simulink model "MPC View 3D"  (R2025b)
settings: Solver=VariableStepAuto  StartTime=0.0  StopTime=15  RelTol=1e-3
values from neighbouring files (symbols this model uses):
  sys_c = ss(A, B, C, D,      'StateName',  {'Angulo (rad)', 'Velocidad (rad/s)'},      'InputName',  {'Torque (Nm)'},      'OutputName', {'Angulo (rad)'})    [Modelo.m]
libraries: simulink x2, autolibshared x1, mpclib x1, sim3dlib x1, sim3dautolib x1
settings Model: Creator=Camilo  LastModifiedBy=Camilo

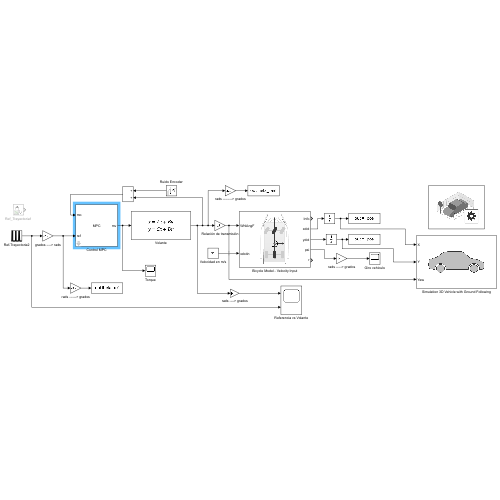
[thumbnail: Simulink's stored preview of the top-level diagram]
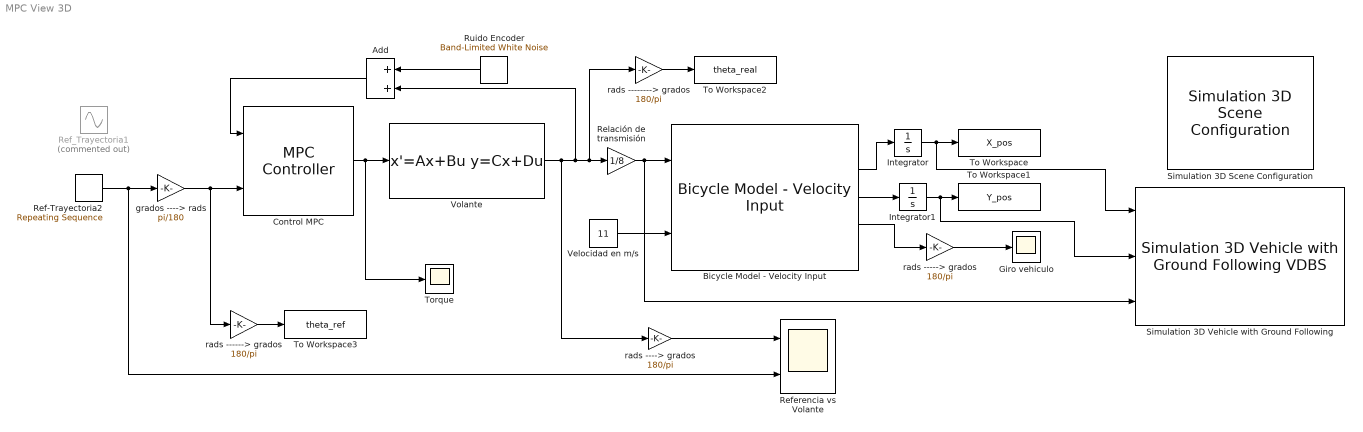
== system MPC View 3D ==
  Add : Sum
  Bicycle Model - Velocity Input : autolibshared/Bicycle Model - Velocity Input  trackMode=Single (bicycle)  inputMode=External longitudinal velocity  frontSteerMode=on  rearSteerMode=off  windMode=off  muMode=off  extFMode=off  extMMode=off  aMode=3  NF=2  NR=2  m=2000  a=1.4  b=1.6  h=0.35  X_o=0  xdot_o=0  CalphaMode=off  sigmaMode=on  w=[1.4,1.4]  Cy_f=12e3  Cy_r=11e3  sigma_f=.1  sigma_r=.1  alpha_f_brk=[-.1 .1]  Cy_f_data=[-9e3 9e3]  alpha_r_brk=[-.1 .1]  Cy_r_data=[-9e3 9e3]  Y_o=0  ydot_o=0  Izz=4000  psi_o=0  r_o=0  Af=2  Cd=.3  Cl=.1  Cpm=.1  beta_w=[0 0.01:0.01:0.3]  Cs=[0 0.01:0.01:0.3]  Cym=[0 1e-6:0.01:0.3]  Pabs=101325  Tair=273  g=9.81  mu=1  xdot_tol=.01  Fznom=5000  Fxtire_sat=1e6  Fytire_sat=1e6  longOff=0  latOff=0  vertOff=0
      settings: LibrarySourceBlock=drivingscenarioandsensors/Bicycle Model - Velocity Input
  Control MPC : mpclib/MPC Controller  SCDEnableBlockLinearizationSpecification=on  mpcobj=mpc1  is_multiple=0  enable_value=0  return_u0=off  updateMPCinCallerWorkspace=on  md_inport=off  mv_inport=off  uref_inport=off  return_cost=off  return_mvseq=off  return_qpstatus=off  return_xseq=off  return_state=off  return_ovseq=off  state_inport=off  umin_inport=off  umax_inport=off  ymin_inport=off  ymax_inport=off  cc_inport=off  ywt_inport=off  uwt_inport=off  duwt_inport=off  rhoeps_inport=off  pm_inport=off  MaximumP=10  HorizonChoice=FixedHorizon  n_ts=0.01  n_p=150  n_mv=1  n_md=0  n_ud=0  n_mo=1  n_uo=0  BlockDataType=double  SampleTimeInherited=off  switch_inport=off
  Giro vehiculo : Scope
      settings: ActiveDisplayYMinimum=-8.075462786158182  ActiveDisplayYMaximum=72.438098994983108
  Integrator : Integrator
  Integrator1 : Integrator
  Ref-Trayectoria2 : simulink/Sources/Repeating Sequence  rep_seq_t=[0, 3, 5, 7, 9, 25]  rep_seq_y=[0, 0, 30, 30, 0, 0]
  Ref_Trayectoria1 : Sin  Commented=on  Amplitude=20  Frequency=0.3  SampleTime=0.01
  Referencia vs Volante : Scope  NumInputPorts=2
      settings: ActiveDisplayYMinimum=-4.394916415083765  ActiveDisplayYMaximum=33.821657379453754  DataLoggingVariableName=ScopeData2
  Relación de transmisión : Gain  Gain=1/8
  Ruido Encoder : simulink/Sources/Band-Limited White Noise  Cov=0.000001  Ts=0.01  seed=[23341]
  Simulation 3D Scene Configuration : sim3dlib/Simulation 3D Scene Configuration  Priority=0  ProjectFormat=Default Scenes  SceneDesc=Double lane change  ProjectName=C:\Program Files\MATLAB\R2025b\toolbox\shared\sim3d_projects\automotive_project_windows\UE\WindowsNoEditor\VehicleSimulation.exe  ScenePath=/Game/Maps/HwStrght  EnableOpenDRIVE=off  vehTagList={'Custom';'Scene Origin';'SimulinkVehicle1'}  vehTag=SimulinkVehicle1  AttachedCameraRelativeTranslation=[0 0 0]  FreeCameraDefaultInitialTranslation=[-6, 0, 2]  AttachedCameraRelativeRotation=[0 0 0]  FreeCameraDefaultInitialRotation=[0, -15, 0]  ViewpointName=Custom  FreeCameraInitialTranslation=[0 0 0]  ViewpointTranslation=[0 0 0]  FreeCameraInitialRotation=[0 0 0]  ViewpointRotation=[0 0 0]  OpVisEn=off  Ts=.01  EnableWindow=on  EnableRemoteAccess=off  EnableWeather=off  SunAzimuth=90  SunAltitude=40.0  EnableGeospatialSun=off  Latitude=0  Longitude=0  Date=2023-01-01  Time=10:30:00  GeoTimeZone=-5.0  SunDaylightSaving=off  wind=1  clouds=10  EnableVolumetricClouds=off  CloudCoverage=0  CloudAltitude=6  fog=0  rain=0  RaindropsEffect=off  SnowDensity=0  EnableGeospatial=off  TilesetSource=Earth terrain  UseTrueOrigin=off  OriginHeight=200  OriginLatitude=40.744652  OriginLongitude=-73.988864  MapStyle=Aerial  AdditionalAssetIDs=[]  UseAdvancedSunSky=off  SolarTime=11  TimeZone=-5  Day=21  Month=9  Year=2022  UseDaylightSavingTime=on  DSTStartDay=10  DSTStartMonth=3  DSTEndDay=3  DSTEndMonth=11  DSTSwitchHour=2  sensorTag=MainCamera1  sensorId=1  sensorName=MainCamera1  mountLoc=Origin  offsetFlag=off  tmountOffset=[0, 0, 0]  rmountOffset=[0, 0, 0]  HorizontalResolution=1280  VerticalResolution=720  HorizontalFOV=60  mountPoint=[0 0 0]  mountOrientation=[0 0 0]  aMode=2  ID=1  GeoTrigger=Inactive  ViewNameList={'Custom'}  ViewTranslationList={'[0 0 0]'}  ViewRotationList={'[0 0 0]'}
      settings: LibrarySourceBlock=vehdynlibsim3dcore/Simulation 3D Scene Configuration
  Simulation 3D Vehicle with Ground Following : sim3dautolib/Simulation 3D Vehicle with Ground Following VDBS  Priority=-1  PassVehMesh=Sedan  MeshPath=/MathWorksAutomotiveContent/Vehicles/Muscle/Meshes/SK_MuscleCar.SK_MuscleCar  TrackWidth=1.9  WheelBase=3  WheelRadius=0.35  VehColor=Blue  CoordinateSystem=SAE  InitialPos=[0, 0, 0]  InitialRot=[0, 0, 0]  ActorName=SimulinkVehicle1  VehLightsControl=off  HeadlightColor=[ 1, 1, 1 ]  HighBeamIntensity=100000  LowBeamIntensity=60000  HighBeamConeAngle=1.22  LowBeamConeAngle=1.22  LeftHeadlightOrientation=[ 0, 0 ]  RightHeadlightOrientation=[ 0, 0 ]  BrakelightIntensity=200  ReverselightIntensity=500  SignallightIntensity=500  SignallightPeriod=1  SignalPulseWidth=50  SampleTime=0.01  ActorType=SimulinkVehicle  ID=1  aMode=2  ActorTag=SimulinkVehicle1  CoordinateScheme=0
      settings: LibrarySourceBlock=vehdynlibsim3d/Simulation 3D Vehicle with Ground Following
  To Workspace : ToWorkspace  VariableName=X_pos  SaveFormat=Timeseries  SampleTime=-1
  To Workspace1 : ToWorkspace  VariableName=Y_pos  SaveFormat=Timeseries  SampleTime=-1
  To Workspace2 : ToWorkspace  VariableName=theta_real  SaveFormat=Timeseries  SampleTime=-1
  To Workspace3 : ToWorkspace  VariableName=theta_ref  SaveFormat=Timeseries  SampleTime=-1
  Torque : Scope
      settings: ActiveDisplayYMinimum=-1  ActiveDisplayYMaximum=1
  Velocidad en m/s : Constant  Value=11
  Volante : StateSpace  A=sys_c.A  B=sys_c.B  C=sys_c.C  D=sys_c.D  InitialCondition=[0;0]
  grados ----> rads : Gain  Gain=pi/180
  rads --------> grados : Gain  Gain=180/pi
  rads ------> grados : Gain  Gain=180/pi
  rads -----> grados : Gain  Gain=180/pi
  rads ----> grados : Gain  Gain=180/pi
  wires:
  Control MPC/1 -> Torque/1, Volante/1
  Volante/1 -> rads ----> grados/1, Add/2, rads --------> grados/1, Relación de transmisión/1
  Ruido Encoder/1 -> Add/1
  Add/1 -> Control MPC/1
  Relación de transmisión/1 -> Simulation 3D Vehicle with Ground Following/3, Bicycle Model - Velocity Input/1
  grados ----> rads/1 -> rads ------> grados/1, Control MPC/2
  Ref-Trayectoria2/1 -> Referencia vs Volante/2, grados ----> rads/1
  Velocidad en m/s/1 -> Bicycle Model - Velocity Input/2
  Bicycle Model - Velocity Input/2 -> Integrator/1
  Bicycle Model - Velocity Input/3 -> Integrator1/1
  Integrator/1 -> Simulation 3D Vehicle with Ground Following/1, To Workspace/1
  Integrator1/1 -> Simulation 3D Vehicle with Ground Following/2, To Workspace1/1
  Bicycle Model - Velocity Input/4 -> rads -----> grados/1
  rads -----> grados/1 -> Giro vehiculo/1
  rads ----> grados/1 -> Referencia vs Volante/1
  rads --------> grados/1 -> To Workspace2/1
  rads ------> grados/1 -> To Workspace3/1
